simulink model "endEffectorControl_WBTv5"  (Simulink 9.1)
settings: Solver=FixedStepDiscrete  StartTime=0.0  StopTime=Config.SIMULATION_TIME  FixedStep=Config.Ts  RelTol=1e-3  EnableMultiTasking=on
InitFcn:
  | initEndEffectorControl
StopFcn:
  | stopEndEffectorControl
undefined symbols (not defined in the file or in its folder): Config, CONFIG, DiscIntNeverNeededParam, GAINS, ROBOT_DOF_FOR_SIMULINK
libraries: WBToolboxLibrary x28, simulink x1
settings Model: SuppressorTable=22 serialization::archive 11 0 6 0 0 0 1 0  Creator=yeshi  LastModifiedBy=yeshi  NumberOfSteps=50
settings DataIOCC: SaveFormat=Dataset
settings DebuggingCC: UnderspecifiedInitializationDetection=Simplified  MergeDetectMultiDrivingBlocksExec=error
settings HardwareCC: ProdBitPerPointer=64  ProdBitPerSizeT=64  ProdBitPerPtrDiffT=64  ProdLargestAtomicFloat=Float  ProdIntDivRoundTo=Zero  ProdEndianess=LittleEndian  ProdWordSize=64  ProdHWDeviceType=Intel->x86-64 (Windows64)
settings ModelReferenceCC: PropagateSignalLabelsOutOfModel=on
settings GRTTargetCC: GeneratePreprocessorConditionals=Disable all  CombineOutputUpdateFcns=on  GRTInterface=off

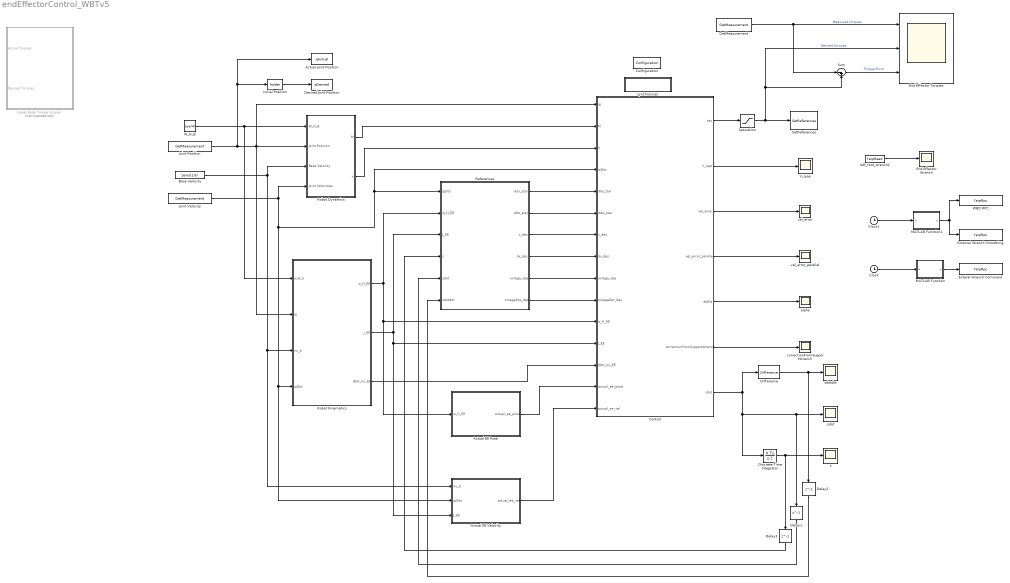
== system endEffectorControl_WBTv5 ==
  Actual EE Pose : MATLAB Function  TreatAsAtomicUnit=on
  Actual EE Velocity : MATLAB Function  TreatAsAtomicUnit=on
  Actual Joint Position : ToWorkspace  VariableName=qActual  SaveFormat=Timeseries  SampleTime=-1
  "Base Velocity " : Constant  Value=zeros(1,6)
  Clock : Clock
  Clock1 : Clock
  Configuration : WBToolboxLibrary/Utilities/Configuration  ConfigSource=Workspace  ConfigObject='WBTConfigRobot'
      settings: SourceProductName=WholeBodyToolbox
  Control : Subsystem
  Delay1 : Delay  DelayLength=1
  Delay2 : Delay  DelayLength=1
  Delay3 : Delay  DelayLength=1
  Desired Joint Position : ToWorkspace  VariableName=qDesired  SaveFormat=Timeseries  SampleTime=-1
  Difference : simulink/Discrete/Difference  ICPrevInput=0.0  OutMin=[]  OutMax=[]  OutDataType=fixdt(1, 16)  OutScaling=2^-10  DoSatur=off
  Discrete-Time Integrator : DiscreteIntegrator  SampleTime=-1  ICPrevOutput=DiscIntNeverNeededParam  ICPrevScaledInput=DiscIntNeverNeededParam
  End Effector Wrench : Scope
  "End Effector Torques " : Scope  NumInputPorts=3
  Exteral Wrench Command : WBToolboxLibrary/Utilities/YarpRpc  risingEdgeTrigger=on  portName=Config.EXT_WRENCH_PORT  rpcCommand=Config.EXT_WRENCH_COMMAND
      settings: SourceProductName=WholeBodyToolbox
  External Wrench Smoothing : WBToolboxLibrary/Utilities/YarpRpc  risingEdgeTrigger=on  portName=Config.EXT_WRENCH_PORT  rpcCommand=Config.EXT_WRENCH_SMOOTHING
      settings: SourceProductName=WholeBodyToolbox
  GetMeasurement : WBToolboxLibrary/States/GetMeasurement  measuredType=Joints Torque
      settings: SourceProductName=WholeBodyToolbox
  "Initial Position " : WBToolboxLibrary/Utilities/holder 
      settings: SourceProductName=WholeBodyToolbox
  Joint Position : WBToolboxLibrary/States/GetMeasurement  measuredType=Joints Position
      settings: SourceProductName=WholeBodyToolbox
  Joint Velocity : WBToolboxLibrary/States/GetMeasurement  measuredType=Joints Velocity
      settings: SourceProductName=WholeBodyToolbox
  MATLAB Function : MATLAB Function  TreatAsAtomicUnit=on
  MATLAB Function1 : MATLAB Function  TreatAsAtomicUnit=on
  References : Subsystem
  Robot Dynamics : Subsystem
  Robot Kinematics : Subsystem
  Saturation : Saturate  UpperLimit=20  LowerLimit=-20
  SetReferences : WBToolboxLibrary/Actuators/SetReferences  controlType=Torque  refSpeed=50  refAcceleration=1000000*(pi/180)
      settings: SourceProductName=WholeBodyToolbox
  Sum : Sum  Inputs=|-+
  Upper Body Torque Scopes : Subsystem  Commented=on
  V_lyap : Scope
  WBD RPC : WBToolboxLibrary/Utilities/YarpRpc  risingEdgeTrigger=on  portName=Config.WBD_RPC_PORT  rpcCommand=Config.WBD_CALIB
      settings: SourceProductName=WholeBodyToolbox
  "W_H_B " : Constant  Value=eye(4)
  alpha : Scope
  correctionFromSupportWrench : Scope
  left_foot_wrench2 : WBToolboxLibrary/Utilities/YarpRead  portName=Ports.EE  signalSize=6  timeout=0.5  blocking=off  timestamp=off  autoconnect=on  errorOnConnection=on
      settings: SourceProductName=WholeBodyToolbox
  s : Scope
  sdot : Scope
  sdotdot : Scope
  synchronizer : Subsystem
      mask Display: disp('SYNCHRONIZER')
  vel_error : Scope
  vel_error_parallel : Scope
  wires:
  Joint Position/1 -> Robot Kinematics/2(qj), Robot Dynamics/2(Joint Position), Control/1(qj), "Initial Position "/1, Actual Joint Position/1
  Joint Velocity/1 -> Robot Dynamics/4(" Joint Velocities "), Actual EE Velocity/2(qjDot), Robot Kinematics/4(qjDot), Control/4(qjDot), References/1(qjDot)
  "W_H_B "/1 -> Robot Kinematics/1(w_H_b), Robot Dynamics/1(W_H_B)
  "Base Velocity "/1 -> Robot Dynamics/3(Base Velocity), Actual EE Velocity/1(nu_b), Robot Kinematics/3(nu_b)
  Robot Kinematics/1(w_H_EE) -> References/2(w_H_EE), Control/11(w_H_EE), Actual EE Pose/1(w_H_EE)
  Control/1(tau) -> Saturation/1
  Robot Kinematics/3(JDot_nu_EE) -> Control/13(JDot_nu_EE)
  Robot Kinematics/2(J_EE) -> Actual EE Velocity/3(J_EE), Control/12(J_EE), References/3(J_EE)
  References/1(ddx_star) -> Control/5(ddx_star)
  Robot Dynamics/2(h) -> Control/3(h)
  References/2(ddw_star) -> Control/6(ddw_star)
  "Initial Position "/1 -> Desired Joint Position/1
  Robot Dynamics/1(M) -> Control/2(M)
  References/5(omega_des) -> Control/9(omega_des)
  References/6(omegaDot_des) -> Control/10(omegaDot_des)
  Actual EE Velocity/1(actual_ee_vel) -> Control/15("actual_ee_vel ")
  References/3(x_des) -> Control/7(x_des)
  References/4(dx_des) -> Control/8(dx_des)
  Actual EE Pose/1(actual_ee_pose) -> Control/14(actual_ee_pose)
  Control/2(V_lyap) -> V_lyap/1
  Control/7(sdot) -> Difference/1, Discrete-Time Integrator/1, Delay1/1, sdot/1
  Discrete-Time Integrator/1 -> s/1, Delay3/1
  left_foot_wrench2/1 -> End Effector Wrench/1
  Saturation/1 -> Sum/2, "End Effector Torques "/2, SetReferences/1  "Desired torques"
  Difference/1 -> Delay2/1, sdotdot/1
  Delay1/1 -> References/5(sdot)
  Delay2/1 -> References/6(sdotdot)
  Delay3/1 -> References/4(s)
  GetMeasurement/1 -> Sum/1, "End Effector Torques "/1  "Measured torques"
  Sum/1 -> "End Effector Torques "/3  "Torque Error"
  Control/5(alpha) -> alpha/1
  Control/6(correctionFromSupportWrench) -> correctionFromSupportWrench/1
  Control/3(vel_error) -> vel_error/1
  Control/4(vel_error_parallel) -> vel_error_parallel/1
  Clock/1 -> MATLAB Function/1(u)
  MATLAB Function/1(y) -> Exteral Wrench Command/1
  MATLAB Function1/1(y) -> WBD RPC/1, External Wrench Smoothing/1
  Clock1/1 -> MATLAB Function1/1(u)

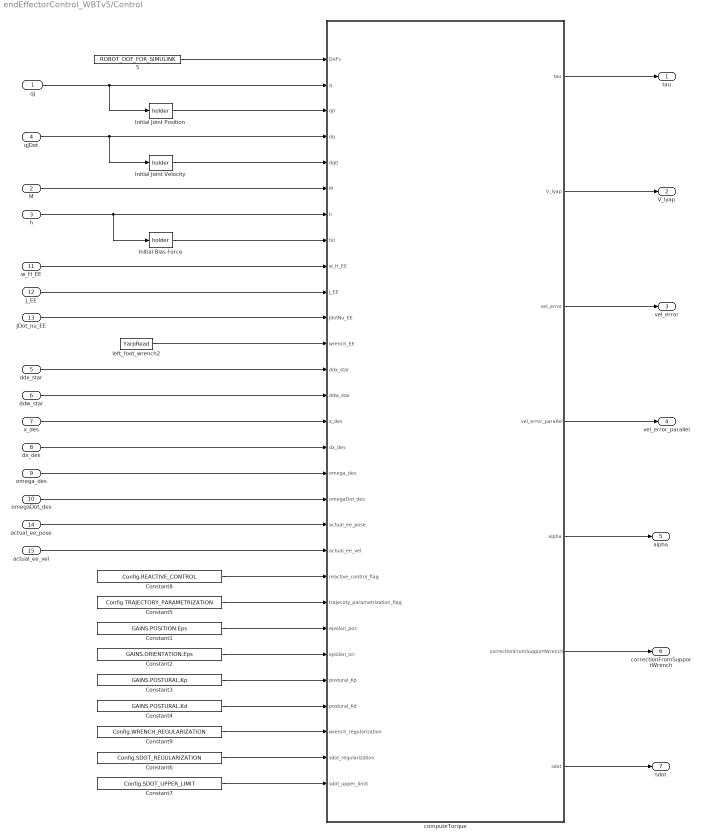
== system endEffectorControl_WBTv5/Control ==
  qj : Inport
  M : Inport  Port=2
  h : Inport  Port=3
  qjDot : Inport  Port=4
  ddx_star : Inport  Port=5
  ddw_star : Inport  Port=6
  x_des : Inport  Port=7
  dx_des : Inport  Port=8
  omega_des : Inport  Port=9
  omegaDot_des : Inport  Port=10
  w_H_EE : Inport  Port=11
  J_EE : Inport  Port=12
  JDot_nu_EE : Inport  Port=13
  actual_ee_pose : Inport  Port=14
  "actual_ee_vel " : Inport  Port=15
  "    5" : Constant  Value=ROBOT_DOF_FOR_SIMULINK
  Constant1 : Constant  Value=GAINS.POSITION.Eps
  Constant2 : Constant  Value=GAINS.ORIENTATION.Eps
  Constant3 : Constant  Value=GAINS.POSTURAL.Kp
  Constant4 : Constant  Value=GAINS.POSTURAL.Kd
  Constant5 : Constant  Value=Config.TRAJECTORY_PARAMETRIZATION
  Constant6 : Constant  Value=Config.SDOT_REGULARIZATION
  Constant7 : Constant  Value=Config.SDOT_UPPER_LIMIT
  Constant8 : Constant  Value=Config.REACTIVE_CONTROL
  Constant9 : Constant  Value=Config.WRENCH_REGULARIZATION  VectorParams1D=off
  Initial Bias Force : WBToolboxLibrary/Utilities/holder 
      settings: SourceProductName=WholeBodyToolbox
  Initial Joint Position : WBToolboxLibrary/Utilities/holder 
      settings: SourceProductName=WholeBodyToolbox
  Initial Joint Velocity : WBToolboxLibrary/Utilities/holder 
      settings: SourceProductName=WholeBodyToolbox
  computeTorque : MATLAB Function  TreatAsAtomicUnit=on
  left_foot_wrench2 : WBToolboxLibrary/Utilities/YarpRead  portName=Ports.EE  signalSize=6  timeout=0.5  blocking=off  timestamp=off  autoconnect=on  errorOnConnection=on
      settings: SourceProductName=WholeBodyToolbox
  tau : Outport
  V_lyap : Outport  Port=2
  vel_error : Outport  Port=3
  vel_error_parallel : Outport  Port=4
  alpha : Outport  Port=5
  correctionFromSupportWrench : Outport  Port=6
  sdot : Outport  Port=7
  wires:
  ddx_star/1 -> computeTorque/13(ddx_star)
  qj/1 -> Initial Joint Position/1, computeTorque/2(q)
  JDot_nu_EE/1 -> computeTorque/11(JdotNu_EE)
  "    5"/1 -> computeTorque/1(DoFs)
  computeTorque/1(tau) -> tau/1
  h/1 -> Initial Bias Force/1, computeTorque/7(h)
  Initial Bias Force/1 -> computeTorque/8(h0)
  Initial Joint Position/1 -> computeTorque/3(q0)
  J_EE/1 -> computeTorque/10(J_EE)
  M/1 -> computeTorque/6(M)
  ddw_star/1 -> computeTorque/14(ddw_star)
  Constant1/1 -> computeTorque/23(epsilon_pos)
  Constant2/1 -> computeTorque/24(epsilon_ori)
  Constant3/1 -> computeTorque/25(postural_Kp)
  Constant4/1 -> computeTorque/26(postural_Kd)
  left_foot_wrench2/1 -> computeTorque/12(wrench_EE)
  Constant5/1 -> computeTorque/22(trajecoty_parametrization_flag)
  omega_des/1 -> computeTorque/17(omega_des)
  omegaDot_des/1 -> computeTorque/18(omegaDot_des)
  "actual_ee_vel "/1 -> computeTorque/20(actual_ee_vel)
  x_des/1 -> computeTorque/15(x_des)
  dx_des/1 -> computeTorque/16(dx_des)
  actual_ee_pose/1 -> computeTorque/19(actual_ee_pose)
  computeTorque/2(V_lyap) -> V_lyap/1
  computeTorque/7(sdot) -> sdot/1
  Initial Joint Velocity/1 -> computeTorque/5(dq0)
  qjDot/1 -> Initial Joint Velocity/1, computeTorque/4(dq)
  Constant6/1 -> computeTorque/28(sdot_regularization)
  Constant7/1 -> computeTorque/29(sdot_upper_limit)
  w_H_EE/1 -> computeTorque/9(w_H_EE)
  Constant8/1 -> computeTorque/21(reactive_control_flag)
  Constant9/1 -> computeTorque/27(wrench_regularization)
  computeTorque/5(alpha) -> alpha/1
  computeTorque/6(correctionFromSupportWrench) -> correctionFromSupportWrench/1
  computeTorque/3(vel_error) -> vel_error/1
  computeTorque/4(vel_error_parallel) -> vel_error_parallel/1

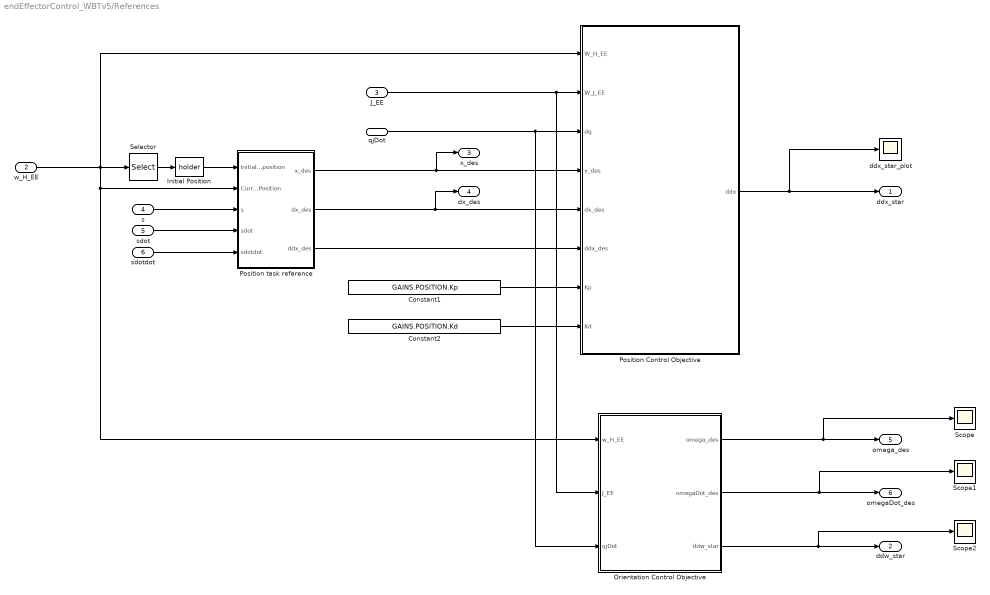
== system endEffectorControl_WBTv5/References ==
  qjDot : Inport
  w_H_EE : Inport  Port=2
  J_EE : Inport  Port=3
  s : Inport  Port=4
  sdot : Inport  Port=5
  sdotdot : Inport  Port=6
  Constant1 : Constant  Value=GAINS.POSITION.Kp
  Constant2 : Constant  Value=GAINS.POSITION.Kd
  "Initial Position " : WBToolboxLibrary/Utilities/holder 
      settings: SourceProductName=WholeBodyToolbox
  Orientation Control Objective : Subsystem
  Position Control Objective : MATLAB Function  TreatAsAtomicUnit=on
  Position task reference : Subsystem
  Scope : Scope
  Scope1 : Scope
  Scope2 : Scope
  Selector : Selector  NumberOfDimensions=2  InputPortWidth=3  IndexOptions=Index vector (dialog),Index vector (dialog)  Indices=[1 2 3],4  OutputSizes=1,1
  ddx_star_plot : Scope
  ddx_star : Outport
  ddw_star : Outport  Port=2
  x_des : Outport  Port=3
  dx_des : Outport  Port=4
  omega_des : Outport  Port=5
  omegaDot_des : Outport  Port=6
  wires:
  J_EE/1 -> Orientation Control Objective/2(J_EE), Position Control Objective/2(W_J_EE)
  Position task reference/1(x_des) -> x_des/1, Position Control Objective/4(x_des)
  Position task reference/2(dx_des) -> dx_des/1, Position Control Objective/5(dx_des)
  Position task reference/3(ddx_des) -> Position Control Objective/6(ddx_des)
  "Initial Position "/1 -> Position task reference/1(Initial position)
  Position Control Objective/1(ddx) -> ddx_star/1, ddx_star_plot/1
  Selector/1 -> "Initial Position "/1
  qjDot/1 -> Orientation Control Objective/3(qjDot), Position Control Objective/3(dq)
  Constant1/1 -> Position Control Objective/7(Kp)
  Constant2/1 -> Position Control Objective/8(Kd)
  Orientation Control Objective/3(ddw_star) -> Scope2/1, ddw_star/1
  w_H_EE/1 -> Position Control Objective/1(W_H_EE), Orientation Control Objective/1(w_H_EE), Position task reference/2(Current Position), Selector/1
  Orientation Control Objective/1(omega_des) -> Scope/1, omega_des/1
  Orientation Control Objective/2(omegaDot_des) -> Scope1/1, omegaDot_des/1
  s/1 -> Position task reference/3(s)
  sdot/1 -> Position task reference/4(sdot)
  sdotdot/1 -> Position task reference/5(sdotdot)

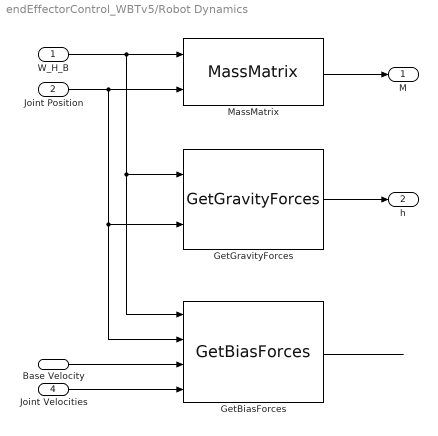
== system endEffectorControl_WBTv5/Robot Dynamics ==
  W_H_B : Inport
  Joint Position : Inport  Port=2
  Base Velocity : Inport  Port=3
  " Joint Velocities " : Inport  Port=4
  GetBiasForces : WBToolboxLibrary/Model/Dynamics/GetBiasForces
      settings: SourceProductName=WholeBodyToolbox
  GetGravityForces : WBToolboxLibrary/Model/Dynamics/GetGravityForces
      settings: SourceProductName=WholeBodyToolbox
  MassMatrix : WBToolboxLibrary/Model/Dynamics/MassMatrix
      settings: SourceProductName=WholeBodyToolbox
  M : Outport
  h : Outport  Port=2
  wires:
  Joint Position/1 -> MassMatrix/2, GetGravityForces/2, GetBiasForces/2
  " Joint Velocities "/1 -> GetBiasForces/4
  GetBiasForces/1 -> ?
  W_H_B/1 -> MassMatrix/1, GetGravityForces/1, GetBiasForces/1
  Base Velocity/1 -> GetBiasForces/3
  MassMatrix/1 -> M/1
  GetGravityForces/1 -> h/1

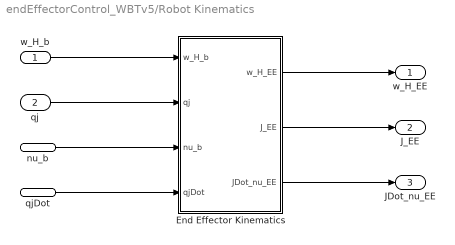
== system endEffectorControl_WBTv5/Robot Kinematics ==
  w_H_b : Inport
  qj : Inport  Port=2
  nu_b : Inport  Port=3
  qjDot : Inport  Port=4
  End Effector Kinematics : Subsystem
  w_H_EE : Outport
  J_EE : Outport  Port=2
  JDot_nu_EE : Outport  Port=3
  wires:
  End Effector Kinematics/1(w_H_EE) -> w_H_EE/1
  End Effector Kinematics/2(J_EE) -> J_EE/1
  End Effector Kinematics/3(JDot_nu_EE) -> JDot_nu_EE/1
  nu_b/1 -> End Effector Kinematics/3(nu_b)
  w_H_b/1 -> End Effector Kinematics/1(w_H_b)
  qj/1 -> End Effector Kinematics/2(qj)
  qjDot/1 -> End Effector Kinematics/4(qjDot)

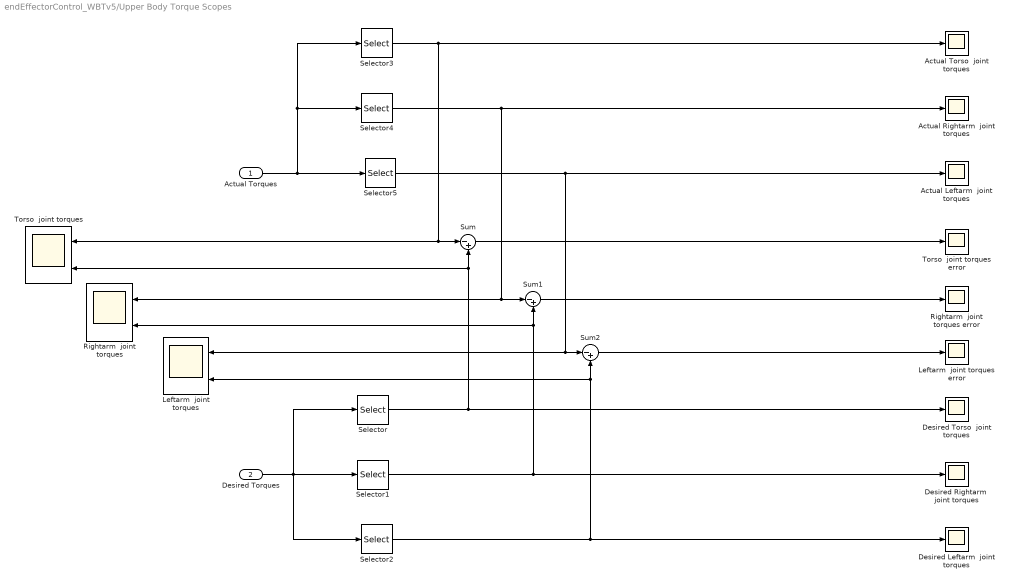
== system endEffectorControl_WBTv5/Upper Body Torque Scopes ==
  Actual Torques : Inport
  Desired Torques : Inport  Port=2
  Actual Leftarm  joint torques : Scope
  Actual Rightarm  joint torques : Scope
  Actual Torso  joint torques : Scope
  Desired Leftarm  joint torques : Scope
  Desired Rightarm  joint torques : Scope
  Desired Torso  joint torques : Scope
  "Leftarm  joint torques " : Scope  NumInputPorts=2
  Leftarm  joint torques error : Scope
  "Rightarm  joint torques " : Scope  NumInputPorts=2
  Rightarm  joint torques error : Scope
  Selector : Selector  InputPortWidth=13  IndexOptions=Index vector (dialog)  Indices=[1:3]  OutputSizes=1
  Selector1 : Selector  InputPortWidth=13  IndexOptions=Index vector (dialog)  Indices=[4 5 6 7 8]  OutputSizes=1
  Selector2 : Selector  InputPortWidth=13  IndexOptions=Index vector (dialog)  Indices=[9 10 11 12 13]  OutputSizes=1
  Selector3 : Selector  InputPortWidth=13  IndexOptions=Index vector (dialog)  Indices=[1:3]  OutputSizes=1
  Selector4 : Selector  InputPortWidth=13  IndexOptions=Index vector (dialog)  Indices=[4 5 6 7 8]  OutputSizes=1
  Selector5 : Selector  InputPortWidth=13  IndexOptions=Index vector (dialog)  Indices=[9 10 11 12 13]  OutputSizes=1
  Sum : Sum  Inputs=|-+
  Sum1 : Sum  Inputs=|-+
  Sum2 : Sum  Inputs=|-+
  "Torso  joint torques " : Scope  NumInputPorts=2
  "Torso  joint torques error " : Scope
  wires:
  Sum/1 -> "Torso  joint torques error "/1
  Sum2/1 -> Leftarm  joint torques error/1
  Selector3/1 -> Actual Torso  joint torques/1, Sum/1, "Torso  joint torques "/1
  Sum1/1 -> Rightarm  joint torques error/1
  Selector4/1 -> Actual Rightarm  joint torques/1, Sum1/1, "Rightarm  joint torques "/1
  Selector/1 -> Desired Torso  joint torques/1, Sum/2, "Torso  joint torques "/2
  Desired Torques/1 -> Selector2/1, Selector/1, Selector1/1
  Actual Torques/1 -> Selector5/1, Selector3/1, Selector4/1
  Selector5/1 -> Actual Leftarm  joint torques/1, Sum2/1, "Leftarm  joint torques "/1
  Selector1/1 -> Sum1/2, "Rightarm  joint torques "/2, Desired Rightarm  joint torques/1
  Selector2/1 -> "Leftarm  joint torques "/2, Sum2/2, Desired Leftarm  joint torques/1

== system endEffectorControl_WBTv5/synchronizer ==
  GAZEBO_SYNCHRONIZER : Subsystem
  Logical Operator : Logic  Operator=NOT  AllPortsSameDT=off  OutDataTypeStr=boolean
  "ON_GAZEBO " : Constant  Value=Config.ON_GAZEBO
  REAL_TIME_SYNC : Subsystem
  To Workspace : ToWorkspace  VariableName=yarp_time  SaveFormat=Structure With Time  SampleTime=-1
  Yarp Clock : WBToolboxLibrary/Utilities/Yarp Clock
      settings: SourceProductName=WholeBodyToolbox
  wires:
  Logical Operator/1 -> REAL_TIME_SYNC/Enable
  "ON_GAZEBO "/1 -> GAZEBO_SYNCHRONIZER/Enable, Logical Operator/1
  Yarp Clock/1 -> To Workspace/1

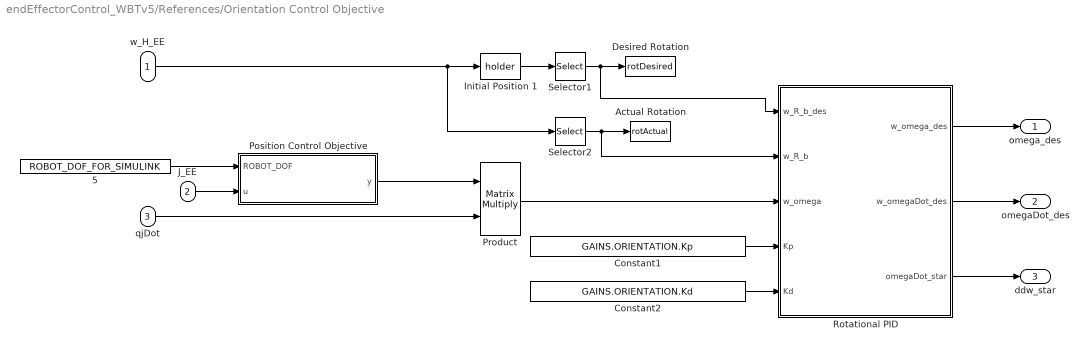
== system endEffectorControl_WBTv5/References/Orientation Control Objective ==
  w_H_EE : Inport
  J_EE : Inport  Port=2
  qjDot : Inport  Port=3
  "    5" : Constant  Value=ROBOT_DOF_FOR_SIMULINK
  Actual Rotation : ToWorkspace  VariableName=rotActual  SaveFormat=Timeseries  SampleTime=-1
  Constant1 : Constant  Value=GAINS.ORIENTATION.Kp
  Constant2 : Constant  Value=GAINS.ORIENTATION.Kd
  Desired Rotation : ToWorkspace  VariableName=rotDesired  SaveFormat=Timeseries  SampleTime=-1
  Initial Position 1 : WBToolboxLibrary/Utilities/holder 
      settings: SourceProductName=WholeBodyToolbox
  Position Control Objective : MATLAB Function  TreatAsAtomicUnit=on
  Product : Product  Multiplication=Matrix(*)
  Rotational PID : MATLAB Function  TreatAsAtomicUnit=on
  Selector1 : Selector  NumberOfDimensions=2  InputPortWidth=4  IndexOptions=Index vector (dialog),Index vector (dialog)  Indices=[1:3],[1:3]  OutputSizes=1,1
  Selector2 : Selector  NumberOfDimensions=2  InputPortWidth=4  IndexOptions=Index vector (dialog),Index vector (dialog)  Indices=[1:3],[1:3]  OutputSizes=1,1
  omega_des : Outport
  omegaDot_des : Outport  Port=2
  ddw_star : Outport  Port=3
  wires:
  Selector2/1 -> Rotational PID/2(w_R_b), Actual Rotation/1
  Rotational PID/3(omegaDot_star) -> ddw_star/1
  Selector1/1 -> Desired Rotation/1, Rotational PID/1(w_R_b_des)
  w_H_EE/1 -> Selector2/1, Initial Position 1/1
  Initial Position 1/1 -> Selector1/1
  Constant1/1 -> Rotational PID/4(Kp)
  Constant2/1 -> Rotational PID/5(Kd)
  qjDot/1 -> Product/2
  Product/1 -> Rotational PID/3(w_omega)
  Position Control Objective/1(y) -> Product/1
  J_EE/1 -> Position Control Objective/2(u)
  "    5"/1 -> Position Control Objective/1(ROBOT_DOF)
  Rotational PID/1(w_omega_des) -> omega_des/1
  Rotational PID/2(w_omegaDot_des) -> omegaDot_des/1

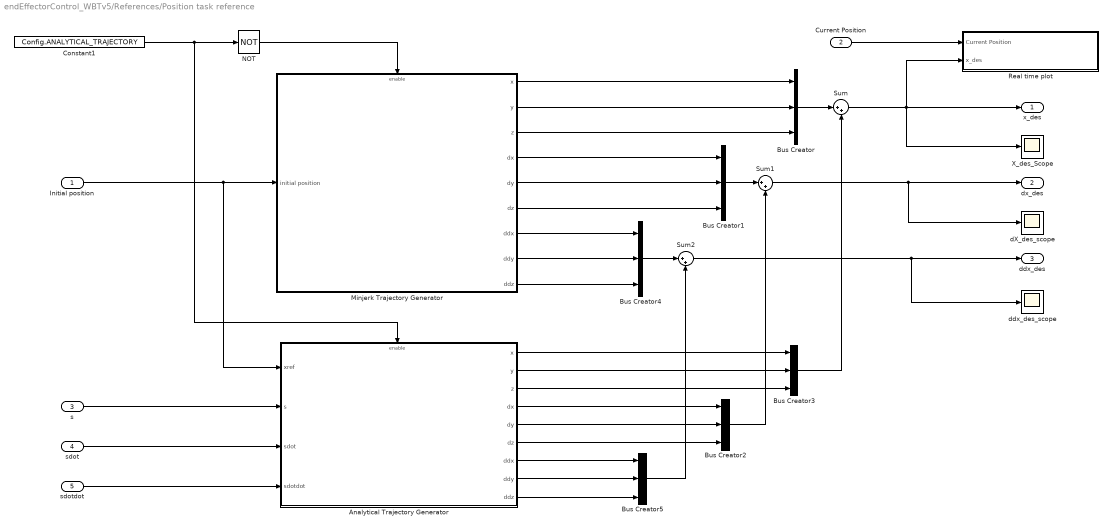
== system endEffectorControl_WBTv5/References/Position task reference ==
  Initial position : Inport
  Current Position : Inport  Port=2
  s : Inport  Port=3
  sdot : Inport  Port=4
  sdotdot : Inport  Port=5
  Analytical Trajectory Generator : Subsystem
  Bus Creator{,1..5} (6 alike) : BusCreator  Inputs=3
  Constant1 : Constant  Value=Config.ANALYTICAL_TRAJECTORY
  Minjerk Trajectory Generator : Subsystem
  NOT : Logic  Operator=NOT  IconShape=distinctive  AllPortsSameDT=off  OutDataTypeStr=boolean
  Real time plot : Subsystem
  Sum : Sum  Inputs=|++
  Sum1 : Sum  Inputs=|++
  Sum2 : Sum  Inputs=|++
  X_des_Scope : Scope
  dX_des_scope : Scope
  ddx_des_scope : Scope
  x_des : Outport
  dx_des : Outport  Port=2
  ddx_des : Outport  Port=3
  wires:
  Minjerk Trajectory Generator/1(x) -> Bus Creator/1
  Minjerk Trajectory Generator/2(y) -> Bus Creator/2
  Minjerk Trajectory Generator/3(z) -> Bus Creator/3
  Minjerk Trajectory Generator/4(dx) -> Bus Creator1/1
  Minjerk Trajectory Generator/5(dy) -> Bus Creator1/2
  Minjerk Trajectory Generator/6(dz) -> Bus Creator1/3
  Minjerk Trajectory Generator/8(ddy) -> Bus Creator4/2
  Minjerk Trajectory Generator/9(ddz) -> Bus Creator4/3
  Bus Creator/1 -> Sum/1
  Sum/1 -> Real time plot/2(x_des), x_des/1, X_des_Scope/1
  Analytical Trajectory Generator/1(x) -> Bus Creator3/1
  Analytical Trajectory Generator/2(y) -> Bus Creator3/2
  Analytical Trajectory Generator/3(z) -> Bus Creator3/3
  Bus Creator3/1 -> Sum/2
  Analytical Trajectory Generator/4(dx) -> Bus Creator2/1
  Analytical Trajectory Generator/5(dy) -> Bus Creator2/2
  Analytical Trajectory Generator/6(dz) -> Bus Creator2/3
  Bus Creator1/1 -> Sum1/1
  Bus Creator2/1 -> Sum1/2
  Sum1/1 -> dX_des_scope/1, dx_des/1
  Minjerk Trajectory Generator/7(ddx) -> Bus Creator4/1
  Analytical Trajectory Generator/7(ddx) -> Bus Creator5/1
  Analytical Trajectory Generator/8(ddy) -> Bus Creator5/2
  Analytical Trajectory Generator/9(ddz) -> Bus Creator5/3
  Bus Creator4/1 -> Sum2/1
  Bus Creator5/1 -> Sum2/2
  Sum2/1 -> ddx_des_scope/1, ddx_des/1
  Constant1/1 -> Analytical Trajectory Generator/Enable, NOT/1
  Current Position/1 -> Real time plot/1(Current Position)
  Initial position/1 -> Analytical Trajectory Generator/1(xref), Minjerk Trajectory Generator/1(initial position)
  s/1 -> Analytical Trajectory Generator/2(s)
  sdot/1 -> Analytical Trajectory Generator/3(sdot)
  sdotdot/1 -> Analytical Trajectory Generator/4(sdotdot)
  NOT/1 -> Minjerk Trajectory Generator/Enable

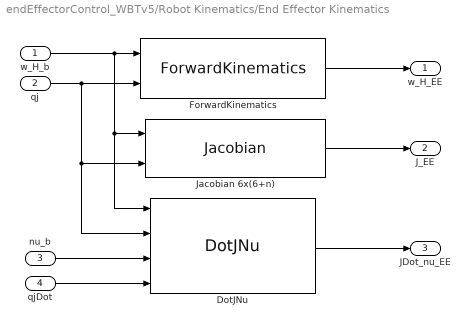
== system endEffectorControl_WBTv5/Robot Kinematics/End Effector Kinematics ==
  w_H_b : Inport
  qj : Inport  Port=2
  nu_b : Inport  Port=3
  qjDot : Inport  Port=4
  DotJNu : WBToolboxLibrary/Model/Jacobians/DotJNu  frameName=Config.EE
      settings: SourceProductName=WholeBodyToolbox
  ForwardKinematics : WBToolboxLibrary/Model/Kinematics/ForwardKinematics  frameName=Config.EE
      settings: SourceProductName=WholeBodyToolbox
  Jacobian 6x(6+n) : WBToolboxLibrary/Model/Jacobians/Jacobian  frameName=Config.EE
      settings: SourceProductName=WholeBodyToolbox
  w_H_EE : Outport
  J_EE : Outport  Port=2
  JDot_nu_EE : Outport  Port=3
  wires:
  qj/1 -> DotJNu/2, Jacobian 6x(6+n)/2, ForwardKinematics/2
  nu_b/1 -> DotJNu/3
  DotJNu/1 -> JDot_nu_EE/1
  ForwardKinematics/1 -> w_H_EE/1
  w_H_b/1 -> DotJNu/1, Jacobian 6x(6+n)/1, ForwardKinematics/1
  Jacobian 6x(6+n)/1 -> J_EE/1
  qjDot/1 -> DotJNu/4

== system endEffectorControl_WBTv5/synchronizer/GAZEBO_SYNCHRONIZER ==
  Enable : EnablePort
  Simulator Synchronizer : WBToolboxLibrary/Utilities/Simulator Synchronizer  period=Config.Ts  serverPortName='/clock/rpc'  clientPortName='/WBT_synchronizer/rpc:o'
      settings: SourceProductName=WholeBodyToolbox

== system endEffectorControl_WBTv5/synchronizer/REAL_TIME_SYNC ==
  Enable : EnablePort
  Real Time Synchronizer : WBToolboxLibrary/Utilities/Real Time Synchronizer  period=Config.Ts
      settings: SourceProductName=WholeBodyToolbox

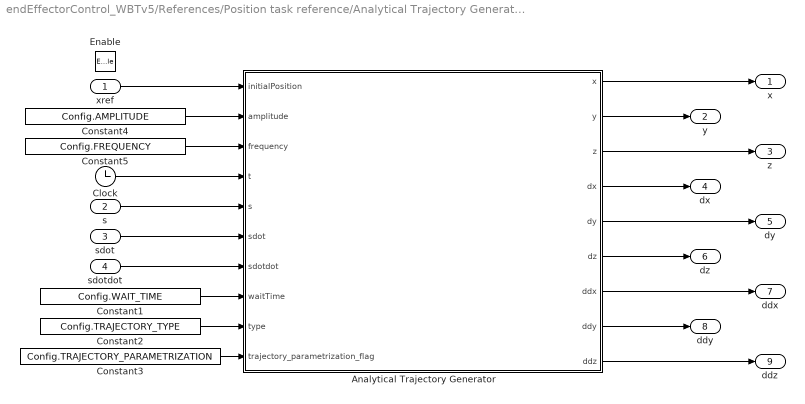
== system endEffectorControl_WBTv5/References/Position task reference/Analytical Trajectory Generator ==
  xref : Inport
  s : Inport  Port=2
  sdot : Inport  Port=3
  sdotdot : Inport  Port=4
  Enable : EnablePort
  Analytical Trajectory Generator : MATLAB Function  TreatAsAtomicUnit=on
  Clock : Clock
  Constant1 : Constant  Value=Config.WAIT_TIME
  Constant2 : Constant  Value=Config.TRAJECTORY_TYPE
  Constant3 : Constant  Value=Config.TRAJECTORY_PARAMETRIZATION
  Constant4 : Constant  Value=Config.AMPLITUDE
  Constant5 : Constant  Value=Config.FREQUENCY
  x : Outport
  y : Outport  Port=2
  z : Outport  Port=3
  dx : Outport  Port=4
  dy : Outport  Port=5
  dz : Outport  Port=6
  ddx : Outport  Port=7
  ddy : Outport  Port=8
  ddz : Outport  Port=9
  wires:
  Analytical Trajectory Generator/5(dy) -> dy/1
  Analytical Trajectory Generator/1(x) -> x/1
  Analytical Trajectory Generator/7(ddx) -> ddx/1
  Analytical Trajectory Generator/8(ddy) -> ddy/1
  Analytical Trajectory Generator/4(dx) -> dx/1
  Analytical Trajectory Generator/2(y) -> y/1
  Analytical Trajectory Generator/9(ddz) -> ddz/1
  Analytical Trajectory Generator/3(z) -> z/1
  Analytical Trajectory Generator/6(dz) -> dz/1
  xref/1 -> Analytical Trajectory Generator/1(initialPosition)
  Constant1/1 -> Analytical Trajectory Generator/8(waitTime)
  s/1 -> Analytical Trajectory Generator/5(s)
  sdot/1 -> Analytical Trajectory Generator/6(sdot)
  sdotdot/1 -> Analytical Trajectory Generator/7(sdotdot)
  Constant2/1 -> Analytical Trajectory Generator/9(type)
  Constant3/1 -> Analytical Trajectory Generator/10(trajectory_parametrization_flag)
  Constant4/1 -> Analytical Trajectory Generator/2(amplitude)
  Constant5/1 -> Analytical Trajectory Generator/3(frequency)
  Clock/1 -> Analytical Trajectory Generator/4(t)

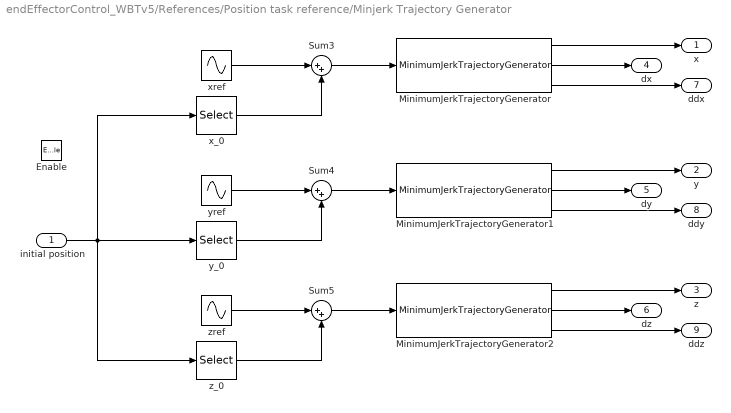
== system endEffectorControl_WBTv5/References/Position task reference/Minjerk Trajectory Generator ==
  initial position : Inport
  Enable : EnablePort
  MinimumJerkTrajectoryGenerator : WBToolboxLibrary/Utilities/MinimumJerkTrajectoryGenerator  externalSettlingTime=off  settlingTime=3  sampleTime=0.01  resetOnSettlingTime=off  firstDerivatives=on  secondDerivatives=on  explicitInitialValue=off
      settings: SourceProductName=WholeBodyToolbox
  MinimumJerkTrajectoryGenerator1 : WBToolboxLibrary/Utilities/MinimumJerkTrajectoryGenerator  externalSettlingTime=off  settlingTime=3  sampleTime=0.01  resetOnSettlingTime=off  firstDerivatives=on  secondDerivatives=on  explicitInitialValue=off
      settings: SourceProductName=WholeBodyToolbox
  MinimumJerkTrajectoryGenerator2 : WBToolboxLibrary/Utilities/MinimumJerkTrajectoryGenerator  externalSettlingTime=off  settlingTime=3  sampleTime=0.01  resetOnSettlingTime=off  firstDerivatives=on  secondDerivatives=on  explicitInitialValue=off
      settings: SourceProductName=WholeBodyToolbox
  Sum3 : Sum  Inputs=|++
  Sum4 : Sum  Inputs=|++
  Sum5 : Sum  Inputs=|++
  x_0 : Selector  InputPortWidth=3  IndexOptions=Index vector (dialog)  Indices=[1]  OutputSizes=1
  xref : Sin  Amplitude=0  SampleTime=0
  y_0 : Selector  InputPortWidth=3  IndexOptions=Index vector (dialog)  Indices=[2]  OutputSizes=1
  yref : Sin  Amplitude=0.075  SampleTime=0
  z_0 : Selector  InputPortWidth=3  IndexOptions=Index vector (dialog)  Indices=[3]  OutputSizes=1
  zref : Sin  Amplitude=0.075  Phase=pi/2  SampleTime=0
  x : Outport
  y : Outport  Port=2
  z : Outport  Port=3
  dx : Outport  Port=4
  dy : Outport  Port=5
  dz : Outport  Port=6
  ddx : Outport  Port=7
  ddy : Outport  Port=8
  ddz : Outport  Port=9
  wires:
  MinimumJerkTrajectoryGenerator/3 -> ddx/1
  MinimumJerkTrajectoryGenerator2/1 -> z/1
  MinimumJerkTrajectoryGenerator1/3 -> ddy/1
  MinimumJerkTrajectoryGenerator2/2 -> dz/1
  MinimumJerkTrajectoryGenerator/2 -> dx/1
  MinimumJerkTrajectoryGenerator/1 -> x/1
  MinimumJerkTrajectoryGenerator1/1 -> y/1
  MinimumJerkTrajectoryGenerator1/2 -> dy/1
  MinimumJerkTrajectoryGenerator2/3 -> ddz/1
  xref/1 -> Sum3/1
  z_0/1 -> Sum5/2
  x_0/1 -> Sum3/2
  Sum3/1 -> MinimumJerkTrajectoryGenerator/1
  initial position/1 -> x_0/1, z_0/1, y_0/1
  y_0/1 -> Sum4/2
  zref/1 -> Sum5/1
  yref/1 -> Sum4/1
  Sum4/1 -> MinimumJerkTrajectoryGenerator1/1
  Sum5/1 -> MinimumJerkTrajectoryGenerator2/1

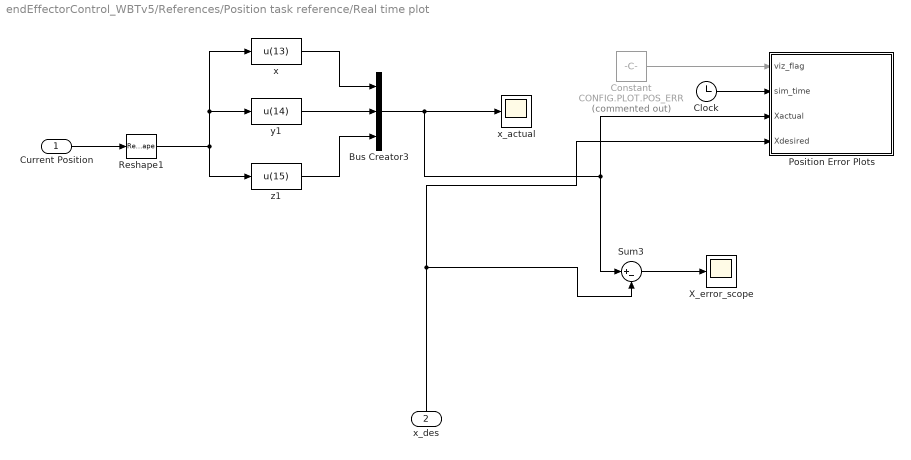
== system endEffectorControl_WBTv5/References/Position task reference/Real time plot ==
  Current Position : Inport
  x_des : Inport  Port=2
  Bus Creator3 : BusCreator  Inputs=3
  Clock : Clock
  Constant : Constant  Commented=on  Value=CONFIG.PLOT.POS_ERR
  "Position Error Plots " : MATLAB Function  TreatAsAtomicUnit=on
  Reshape1 : Reshape
  Sum3 : Sum  Inputs=|+-
  X_error_scope : Scope
  x : Fcn  Expr=u(13)
  x_actual : Scope
  y1 : Fcn  Expr=u(14)
  z1 : Fcn  Expr=u(15)
  wires:
  x_des/1 -> Sum3/2, "Position Error Plots "/4(Xdesired)
  Current Position/1 -> Reshape1/1
  Reshape1/1 -> x/1, y1/1, z1/1
  x/1 -> Bus Creator3/1
  y1/1 -> Bus Creator3/2
  z1/1 -> Bus Creator3/3
  Clock/1 -> "Position Error Plots "/2(sim_time)
  Bus Creator3/1 -> x_actual/1, Sum3/1, "Position Error Plots "/3(Xactual)
  Constant/1 -> "Position Error Plots "/1(viz_flag)
  Sum3/1 -> X_error_scope/1

== matlab function References/Position Control Objective ==
  data: W_H_EE input double; ddx output double; W_J_EE input double; dq input double; x_des input double; dx_des input double; ddx_des input double; Kp input double; Kd input double
function ddx = controlObjective(W_H_EE,W_J_EE,dq,x_des,dx_des,ddx_des,Kp,Kd)
   
    x  = W_H_EE(1:3,4)-x_des;
    dx = W_J_EE(1:3,7:end)*dq-dx_des;
    
    ddx = ddx_des-Kp*x-Kd*dx; 

end

== matlab function Control/computeTorque ==
  data: DoFs input double; q input double; q0 input double; dq input double; dq0 input double; M input double; h input double; h0 input double; w_H_EE input double; J_EE input double; JdotNu_EE input double; wrench_EE input double; ddx_star input double; tau output double; ddw_star input double; x_des input double; dx_des input double; omega_des input double; omegaDot_des input double; actual_ee_pose input double; actual_ee_vel input double; reactive_control_flag input double; trajecoty_parametrization_flag input double; epsilon_pos input double; epsilon_ori input double; postural_Kp input double; postural_Kd input double; wrench_regularization input double; V_lyap output double; vel_error output double; vel_error_parallel output double; alpha output double; correctionFromSupportWrench output double; sdot output double; sdot_regularization input double; sdot_upper_limit input double
 function [tau,V_lyap,vel_error,vel_error_parallel, alpha,correctionFromSupportWrench,sdot] = computeTorque(DoFs,q,q0,dq,dq0,M,h,h0,...
                                                                             w_H_EE,J_EE,JdotNu_EE,...
                                                                             wrench_EE,...
                                                                             ddx_star,ddw_star,x_des,dx_des,omega_des,omegaDot_des,...
                                                                             actual_ee_pose,actual_ee_vel,...
                                                                             reactive_control_flag, trajecoty_parametrization_flag,...
                                                                             epsilon_pos,epsilon_ori,postural_Kp,postural_Kd,...
                                                                             wrench_regularization, sdot_regularization, sdot_upper_limit)

    Dofs = size(DoFs,1);
    
    Sb = zeros(Dofs,6);
    Ss = eye(Dofs);
    S = [Sb Ss]';
    
    %% Initialize zero torques
    tau = zeros(Dofs,1);
        
    %% Initialize svalue
    sdot = 0;
    
    %% compute J^T*f_ext
    EE_ext_wrench = J_EE(:,7:end)'*wrench_EE;

    ddX_star = [ddx_star' ddw_star']';
    
    %% Pose and velocity
    desired_ee_pose = [x_des; omega_des];
    ee_pose_tilde   = actual_ee_pose - desired_ee_pose;
    
    desired_ee_vel  = [dx_des; omegaDot_des];
    ee_vel_tilde    = actual_ee_vel - desired_ee_vel;
    
    %% Velocity error
    vel_error       = actual_ee_vel - desired_ee_vel;
    
    %% Lyapunov function
    %% TODO: Use and check the gain matrices have any effect
    Kd_lyap = 1;
    Kp_lyap = 1;
    
    V_lyap = 0.5*Kd_lyap*transpose(ee_vel_tilde)*ee_vel_tilde;
    V_lyap = V_lyap + 0.5*Kp_lyap*transpose(ee_pose_tilde)*ee_pose_tilde;
    
    %% Wrench decomposition
    vel_error_parallel = vel_error/(norm(vel_error) + wrench_regularization);
    alpha = 0; %% initialization
    correctionFromSupportWrench = zeros(6,1);
    
    if (~trajecoty_parametrization_flag)
        
        %% Compute composite matrices
        JeeMinv = J_EE(:,7:end)/M(7:end,7:end);
        Delta = JeeMinv;
        DeltaPinvDamped = pinvDamped(Delta,epsilon_pos);
        
        alpha         = (transpose(vel_error)*wrench_EE)/(norm(vel_error) + wrench_regularization);
        
        if (alpha < 0)
                correctionFromSupportWrench = alpha * vel_error_parallel;
        end
        
        if (reactive_control_flag)
            %% Update desired dynamics
            ddX_star = ddX_star + correctionFromSupportWrench;
        end
        
        %% Compute robot torques
        tau_pri = DeltaPinvDamped*(ddX_star - JdotNu_EE + (J_EE(:,7:end)/M(7:end,7:end))*h(7:end) - (J_EE(:,7:end)/M(7:end,7:end))*(EE_ext_wrench));
        
        nullspace = eye(size(Delta,2)) - DeltaPinvDamped*Delta;
        
        tau_null = S'*h - postural_Kp*(q-q0) - postural_Kd*(dq-dq0);
        
        tau = tau_pri + nullspace*tau_null;
        
    else
        
        %% Compute composite matrices
        JeeMinv = J_EE(:,7:end)/M(7:end,7:end);
        Delta = JeeMinv;
        DeltaPinvDamped = pinvDamped(Delta,epsilon_pos);
        Gamma = JeeMinv*J_EE(:,7:end)';
        ext_wrench = Gamma*wrench_EE;
        Lambda = JdotNu_EE - JeeMinv*h(7:end);
        Beta = ee_pose_tilde - ddX_star;
        
        %% Compute robot torques
        tau_pri = -DeltaPinvDamped*(Lambda + Beta + ee_vel_tilde);
        
        nullspace = eye(size(Delta,2)) - DeltaPinvDamped*Delta;
        
        %%Second Approach
        tau_null = S'*h - postural_Kp*(q-q0) - postural_Kd*(dq-dq0);
    
        tau = tau_pri + nullspace*tau_null;
        
% %         sdot = max(1, (actual_ee_vel'*ext_wrench)/(desired_ee_vel'*ext_wrench));
        sdot = min(sdot_upper_limit, max(1, ((actual_ee_vel'*ext_wrench)*(desired_ee_vel'*ext_wrench))/((desired_ee_vel'*ext_wrench)^2 + sdot_regularization)));
    end
    
end

== matlab function References/Position task reference/Real time plot/Position Error Plots  ==
  data: viz_flag input double; sim_time input double; Xactual input double; Xdesired input double
function positionErrorPlots(viz_flag,sim_time,Xactual,Xdesired)
%#codegen

coder.extrinsic('animatedline')
coder.extrinsic('addpoints')
coder.extrinsic('legend')
coder.extrinsic('clearpoints')

if(viz_flag ~= 0)
    
    Xerror = Xactual - Xdesired;
    curve_position_error = animatedline('LineWidth',0.1,'Marker','+');

    if(sim_time == 0)
    
        clf;
        close;
    
        fig1 = figure;
        view(177,15); hold on;
        grid on;
        xlabel('x');
        ylabel('y');
        zlabel('z');
        title('Position Error'); hold on;
% %         axis([-0.3 0.3 -0.3 0.3 -0.3 0.3]);
       
    end
    
    figure(1);
    addpoints(curve_position_error,Xerror(1),Xerror(2),Xerror(3));
    drawnow;
    
end

end

== matlab function References/Orientation Control Objective/Rotational PID ==
  data: w_omega_des output double; w_omegaDot_des output double; w_R_b_des input double; w_R_b input double; w_omega input double; omegaDot_star output double; Kp input double; Kd input double
function [w_omega_des,w_omegaDot_des,omegaDot_star]= rotPID(w_R_b_des,w_R_b,w_omega,Kp,Kd)

    w_omega_des = [0;0;0];
    w_omegaDot_des = [0;0;0];
    
% %     omegaDot_star = rotationalPID(w_R_b,w_omega,w_R_b_des,w_omega_des,w_omegaDot_des,Kp,Kd);
    omegaDot_star = rotationalPID_acceleration(w_R_b,w_omega,w_R_b_des,w_omega_des,w_omegaDot_des,Kp,Kd);
end

== matlab function References/Orientation Control Objective/Position Control Objective ==
  data: ROBOT_DOF input double; y output double; u input double
function y = jacobianReordering(ROBOT_DOF, u)
   y = u(4:6,7:6+size(ROBOT_DOF,1));
end

== matlab function References/Position task reference/Analytical Trajectory Generator/Analytical Trajectory Generator ==
  data: x output double; initialPosition input double; amplitude input double; frequency input double; t input double; s input double; sdot input double; sdotdot input double; y output double; z output double; dx output double; dy output double; dz output double; ddx output double; ddy output double; ddz output double; waitTime input double; type input double; trajectory_parametrization_flag input double
function [x,y,z,dx,dy,dz,ddx,ddy,ddz] = fcn(initialPosition, amplitude, frequency, t, s, sdot, sdotdot, waitTime, type, trajectory_parametrization_flag)

    persistent svalue;
    persistent sdotvalue;
    persistent sdotdotvalue;
    
    omega = 2*pi*frequency;
        
    %% Position
    x = initialPosition(1);
    y = initialPosition(2);
    z = initialPosition(3);
             
    %% Velocity
    dx = 0;
    dy = 0;
    dz = 0;
    
    %% Acceleration
    ddx = 0;
    ddy = 0;
    ddz = 0;
    
    if (~trajectory_parametrization_flag)
        svalue       = t;
        sdotvalue    = 1;
        sdotdotvalue = 1;
    else
        svalue       = s;
        sdotvalue    = sdot;
        sdotdotvalue = sdotdot;
    end
        
    if (svalue > waitTime)
        
        currentTime = svalue - waitTime;
        
       if (type == 0)
           
           %% Position
            x = amplitude*sin(omega*currentTime) + initialPosition(1);
            y = amplitude*0 + initialPosition(2);
            z = amplitude*0 + initialPosition(3);
    
            %% Velocity
            dx = amplitude*omega*cos(omega*currentTime)*sdotvalue;
            dy = 0;
            dz = 0;
    
            %% Acceleration
            ddx = -amplitude*(omega*omega)*sin(omega*currentTime)*(sdotvalue*sdotvalue) + amplitude*omega*cos(omega*currentTime)*sdotdotvalue;
            ddy = 0;
            ddz = 0;

       elseif (type == 1)
           
           %% Position
            x = amplitude*0 + initialPosition(1);
            y = amplitude*sin(omega*currentTime) + initialPosition(2);
            z = amplitude*0 + initialPosition(3) ;
    
            %% Velocity
            dx = 0;
            dy = amplitude*omega*cos(omega*currentTime)*sdotvalue;
            dz = 0;
    
            %% Acceleration
            ddx = 0;
            ddy = -amplitude*(omega*omega)*sin(omega*currentTime)*(sdotvalue*sdotvalue) + amplitude*omega*cos(omega*currentTime)*sdotdotvalue;
            ddz = 0;
           
       elseif (type == 2)
           
            %% Position
            x = amplitude*0 + initialPosition(1);
            y = amplitude*0 + initialPosition(2);
            z = amplitude*sin(omega*currentTime) + initialPosition(3) ;
    
            %% Velocity
            dx = 0;
            dy = 0;
            dz = amplitude*omega*cos(omega*currentTime)*sdotvalue;
    
            %% Acceleration
            ddx = 0;
            ddy = 0;
            ddz = -amplitude*(omega*omega)*sin(omega*currentTime)*(sdotvalue*sdotvalue) + amplitude*omega*cos(omega*currentTime)*sdotdotvalue;
            
       elseif (type == 3) %yz
           
            %% Position
            x = amplitude*0 + initialPosition(1);
            y = amplitude*cos(omega*currentTime) + initialPosition(2) - amplitude;
            z = amplitude*sin(omega*currentTime) + initialPosition(3) + amplitude*sin(omega*currentTime + pi/2) + amplitude*cos(omega*currentTime + pi);
    
            %% Velocity
            dx = 0;
            dy = -amplitude*omega*sin(omega*currentTime)*sdotvalue;
            dz =  amplitude*omega*cos(omega*currentTime)*sdotvalue + amplitude*omega*cos(omega*currentTime)*sdotvalue - amplitude*omega*sin(omega*currentTime)*sdotvalue;
    
            %% Acceleration
            ddx = 0;
            ddy = -amplitude*(omega*omega)*cos(omega*currentTime)*(sdotvalue*sdotvalue) - amplitude*omega*sin(omega*currentTime)*sdotdotvalue;
            ddz = -amplitude*(omega*omega)*sin(omega*currentTime)*(sdotvalue*sdotvalue) + amplitude*omega*cos(omega*currentTime)*sdotdotvalue...
                  -amplitude*(omega*omega)*sin(omega*currentTime)*(sdotvalue*sdotvalue) + amplitude*omega*cos(omega*currentTime)*sdotdotvalue...
                  -amplitude*(omega*omega)*cos(omega*currentTime)*(sdotvalue*sdotvalue) - amplitude*omega*sin(omega*currentTime)*sdotdotvalue;
       
       elseif (type == 4) %xz
           
            %% Position
            x = amplitude*cos(omega*currentTime) + initialPosition(1) - amplitude;
            y = amplitude*0 + initialPosition(2);
            z = amplitude*sin(omega*currentTime) + initialPosition(3) + amplitude*sin(omega*currentTime + pi/2) + amplitude*cos(omega*currentTime + pi);
    
            %% Velocity
            dx = -amplitude*omega*sin(omega*currentTime)*sdotvalue;
            dy = 0;
            dz =  amplitude*omega*cos(omega*currentTime)*sdotvalue + amplitude*omega*cos(omega*currentTime)*sdotvalue - amplitude*omega*sin(omega*currentTime)*sdotvalue;
    
            %% Acceleration
            ddx = -amplitude*(omega*omega)*cos(omega*currentTime)*(sdotvalue*sdotvalue) - amplitude*omega*sin(omega*currentTime)*sdotdotvalue;
            ddy = 0;
            ddz = -amplitude*(omega*omega)*sin(omega*currentTime)*(sdotvalue*sdotvalue) + amplitude*omega*cos(omega*currentTime)*sdotdotvalue...
                  -amplitude*(omega*omega)*sin(omega*currentTime)*(sdotvalue*sdotvalue) + amplitude*omega*cos(omega*currentTime)*sdotdotvalue...
                  -amplitude*(omega*omega)*cos(omega*currentTime)*(sdotvalue*sdotvalue) - amplitude*omega*sin(omega*currentTime)*sdotdotvalue;

       elseif (type == 5) %xy
           
            %% Position
            x = amplitude*cos(omega*currentTime) + initialPosition(1) - amplitude;
            y = amplitude*sin(omega*currentTime) + initialPosition(2) + amplitude*sin(omega*currentTime + pi/2) + amplitude*cos(omega*currentTime + pi);
            z = amplitude*0 + initialPosition(3);
    
            %% Velocity
            dx = -amplitude*omega*sin(omega*currentTime)*sdotvalue;
            dy = amplitude*omega*cos(omega*currentTime)*sdotvalue + amplitude*omega*cos(omega*currentTime)*sdotvalue - amplitude*omega*sin(omega*currentTime)*sdotvalue;
            dz = 0;
    
            %% Acceleration
            ddx = -amplitude*(omega*omega)*cos(omega*currentTime)*(sdotvalue*sdotvalue) - amplitude*omega*sin(omega*currentTime)*sdotdotvalue;
            ddy = -amplitude*(omega*omega)*sin(omega*currentTime)*(sdotvalue*sdotvalue) + amplitude*omega*cos(omega*currentTime)*sdotdotvalue...
                  -amplitude*(omega*omega)*sin(omega*currentTime)*(sdotvalue*sdotvalue) + amplitude*omega*cos(omega*currentTime)*sdotdotvalue...
                  -amplitude*(omega*omega)*cos(omega*currentTime)*(sdotvalue*sdotvalue) - amplitude*omega*sin(omega*currentTime)*sdotdotvalue;
            ddz = 0;
            
       end
           
    end
end

== matlab function Actual EE Velocity ==
  data: nu_b input double; actual_ee_vel output double; qjDot input double; J_EE input double
function actual_ee_vel = fcn(nu_b, qjDot,J_EE)

    actual_ee_vel = J_EE*[nu_b; qjDot];

end

== matlab function Actual EE Pose ==
  data: w_H_EE input double; actual_ee_pose output double
function actual_ee_pose = fcn(w_H_EE)

    ee_position    = w_H_EE(1:3,4);
    
    ee_rotMatrix   = w_H_EE(1:3,1:3);
    ee_oriEuler    = rotm2euler(ee_rotMatrix);
    
    actual_ee_pose = [ee_position; ee_oriEuler]; 

end

== matlab function MATLAB Function ==
  data: u input double; y output double
function y = fcn(u)

    y = 0;
    if (u > 6 && u < 6.02)
        y = 1;
    end

end

== matlab function MATLAB Function1 ==
  data: u input double; y output double
function y = fcn(u)

    y = 0;
    if (u > 0 && u < 0.02)
        y = 1;
    end

end
